simulink model "prelab6model"  (R2024a)
settings: Solver=VariableStepAuto  StartTime=0.0  StopTime=10.0  RelTol=1e-3
values from neighbouring files (symbols this model uses):
  tau_p = 0.0073    [lab6main.m]    (also in lab6report.m = 0.007)
  tau_z = 0.068    [lab6main.m]    (also in lab6report.m = 0.07)
settings Model: Creator=xinchen  LastModifiedBy=xinchen

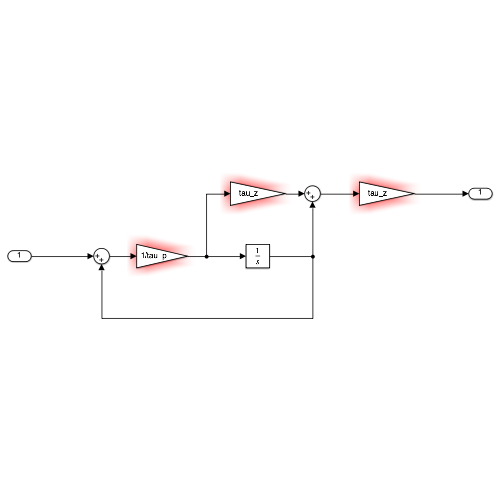
[thumbnail: Simulink's stored preview of the top-level diagram]
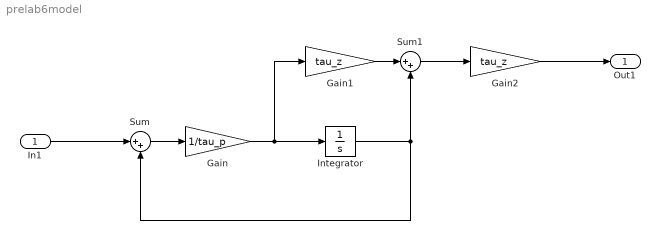
== system prelab6model ==
  In1 : Inport
  Gain : Gain  Gain=1/tau_p
  Gain1 : Gain  Gain=tau_z
  Gain2 : Gain  Gain=tau_z
  Integrator : Integrator
  Sum : Sum  Inputs=|++
  Sum1 : Sum  Inputs=|++
  Out1 : Outport
  wires:
  In1/1 -> Sum/1
  Sum/1 -> Gain/1
  Gain/1 -> Gain1/1, Integrator/1
  Integrator/1 -> Sum1/2, Sum/2
  Gain1/1 -> Sum1/1
  Sum1/1 -> Gain2/1
  Gain2/1 -> Out1/1
